simulink model "MatlabCode-Thermosys"  (R2014a)
settings: Solver=ode23tb  StartTime=0.0  StopTime=1000  RelTol=1e-3
libraries: thermosys x4
settings Model: CovSFcnEnable=on  Creator=garrow2  LastModifiedBy=VILLAVI1
settings DataIOCC: LimitDataPoints=off  SaveFormat=StructureWithTime
settings DebuggingCC: MergeDetectMultiDrivingBlocksExec=error  SolverPrmCheckMsg=none  FrameProcessingCompatibilityMsg=error
settings HardwareCC: ProdBitPerPointer=64  ProdLargestAtomicFloat=Float  ProdIntDivRoundTo=Zero  ProdEndianess=LittleEndian  ProdHWDeviceType=Specified
settings ModelReferenceCC: PropagateSignalLabelsOutOfModel=on

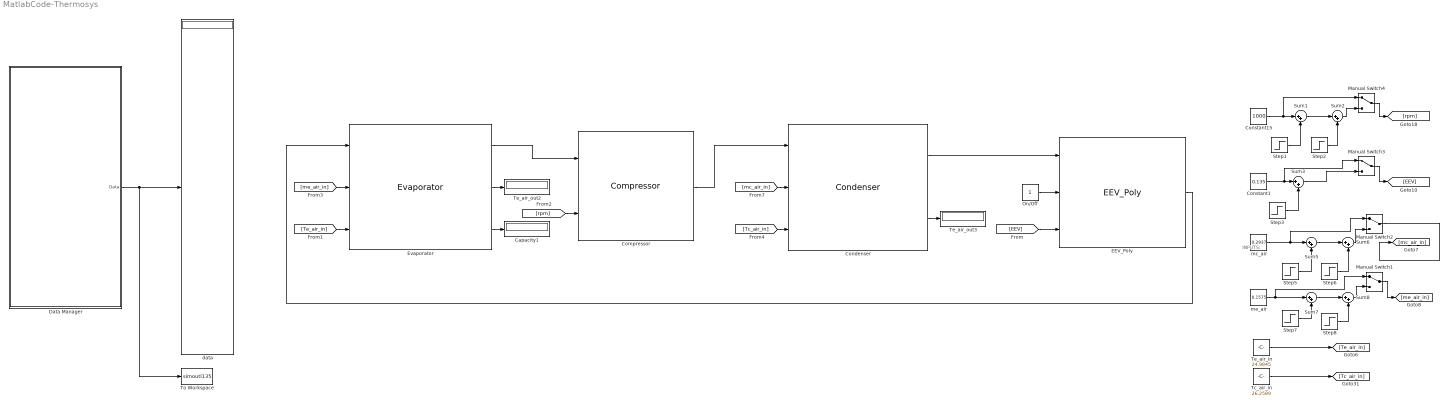
== system MatlabCode-Thermosys ==
  note: INPUTS:
  Capacity1 : Display
  Compressor : thermosys/Components/Compressor  Vk=3.042e-5  HTC=25  CFile=CompProp  REFR=R134a  Pk_ri=279.1497  Pk_ro=968.3655  Tk_ri=19.9747  Tk_ro=61.4005  mdot=0.0062  rpm=1500  IODS=Text
  Condenser : thermosys/Components/Condenser  Dh=8.1026e-3  L=10.6895  N=1  Ac_air=.089798964  As_air=2.792665382  As_ref=0.274993  Ac_ref=5.15631e-5  M_wall=4.65636  Cp_wall=.0467  PAF_TP=1  PAF_SH=0.5  PAF_SC=1  PAF_AIR=1.2  REFR=R134a  MFR=0.0062  PREF=968  RIT=61.8  ROE=250  MFA=0.2937  AIT=25  IODS=Text
  Constant1 : Constant  Value=0.135
  Constant15 : Constant  Value=1000
  Data Manager : Subsystem  AncestorBlock=thermosys/Support Components/Data Manager  mask{null=0}
      mask init:
      | set_param(gcb, 'LinkStatus', 'inactive')    % disable the library link
      settings: OpenFcn=data_manager
      mask Display: str ='Compressor/P_out_ref\nCompressor/h_out_ref\nCompressor/mdot_out_ref\nCondenser/P_out_ref\nCondenser/h_out_ref\nCondenser/T_out_ref\nCondenser/mdot_out_ref\nCondenser/T_out_air\nCondenser/T_wall1\nCondenser/T_wall2\nCondenser/T_wall3\nCondenser/Zeta1\nCondenser/Zeta2\nCondenser/Zeta3\nCondenser/Mass\nEEV_Poly/P_out_ref\nEEV_Poly/h_out_ref\nEEV_Poly/mdot_out_ref\nEvaporator/P_out_ref\nEvaporator/h_out_ref\nEvaporator/T_out_ref\nEvaporator/mdot_out_ref\nEvaporator/T_out_air\nEvaporator/T_wall1\nEvaporator/T_wall2\nEvaporator/Zeta1\nEvaporator/Zeta2\nEvaporator/Mass\nEvaporator/Cool_Cap'; fprintf(str)
  EEV_Poly : thermosys/Components/EEV_Poly  cv_max=4e-5  stroke_fraction=[0:0.1:1]  cv_fraction=[0:0.1:1].*(2.0-[0:0.1:1])  IODS=Text  REFR=R134a  p1=-2e-13  p2=5.6e-13  p3=-5.8e-13  p4=2.6e-13  p5=-1  p6=2  p7=1.1e-16
  Evaporator : thermosys/Components/Evaporator  Dh=8.126e-3  L=11.45794  N=1  Ac_air=.058384399  As_air=3.068019456  As_ref=.0291662649  Ac_ref=5.15631e-5  M_wall=2.7438213  Cp_wall=0.48772265  PAF_TP=1  PAF_SH=2  PAF_AIR=1.1  REFR=R134a  MFR=0.0062  PREF=295.3  HREFIN=245  TRO=12  MFA=0.105  AIT=25  IODS=Text
  Manual Switch{1..4} (4 alike) : ManualSwitch
  On/Off : Constant
  Step1 : Step  Time=100  After=-1500  SampleTime=0
  Step2 : Step  Time=500  After=1500  SampleTime=0
  Step3 : Step  Time=100  After=-0.06  SampleTime=0
  Step5 : Step  Time=100  After=-0.2937  SampleTime=0
  Step6 : Step  Time=500  After=0.2937  SampleTime=0
  Step7 : Step  Time=100  After=-0.105  SampleTime=0
  Step8 : Step  Time=500  After=0.105  SampleTime=0
  Sum{1..3,5..8} (7 alike) : Sum  Inputs=|++
  Tc_air_in : Constant  Value=26.2589
  Te_air_in : Constant  Value=24.9845
  Te_air_out2 : Display
  Te_air_out3 : Display
  To Workspace : ToWorkspace  VariableName=simoutl135  SaveFormat=Timeseries  SampleTime=-1
  data : Display
  mc_air : Constant  Value=0.2937
  me_air : Constant  Value=0.1575
  wires:
  [EEV] -> EEV_Poly/3
  On/Off/1 -> EEV_Poly/2
  [Tc_air_in] -> Condenser/3
  [mc_air_in] -> Condenser/2
  [rpm] -> Compressor/2
  [me_air_in] -> Evaporator/2
  [Te_air_in] -> Evaporator/3
  Evaporator/2 -> Te_air_out2/1
  Evaporator/3 -> Capacity1/1
  Condenser/2 -> Te_air_out3/1
  Evaporator/1 -> Compressor/1
  Compressor/1 -> Condenser/1
  Condenser/1 -> EEV_Poly/1
  EEV_Poly/1 -> Evaporator/1
  Tc_air_in/1 -> [Tc_air_in]
  Te_air_in/1 -> [Te_air_in]
  Constant15/1 -> Manual Switch4/1, Sum1/1
  Step1/1 -> Sum1/2
  Sum1/1 -> Sum2/1
  Step2/1 -> Sum2/2
  Constant1/1 -> Manual Switch3/1, Sum3/1
  Step3/1 -> Sum3/2
  Step5/1 -> Sum5/2
  Step6/1 -> Sum6/2
  mc_air/1 -> Manual Switch2/1, Sum5/1
  Sum5/1 -> Sum6/1
  Step7/1 -> Sum7/2
  Step8/1 -> Sum8/2
  Sum7/1 -> Sum8/1
  me_air/1 -> Manual Switch1/1, Sum7/1
  Sum6/1 -> Manual Switch2/2
  Data Manager/1(Data) -> To Workspace/1, data/1
  Sum8/1 -> Manual Switch1/2
  Manual Switch1/1 -> [me_air_in]
  Manual Switch2/1 -> [mc_air_in]
  Manual Switch3/1 -> [EEV]
  Manual Switch4/1 -> [rpm]
  Sum2/1 -> Manual Switch4/2
  Sum3/1 -> Manual Switch3/2

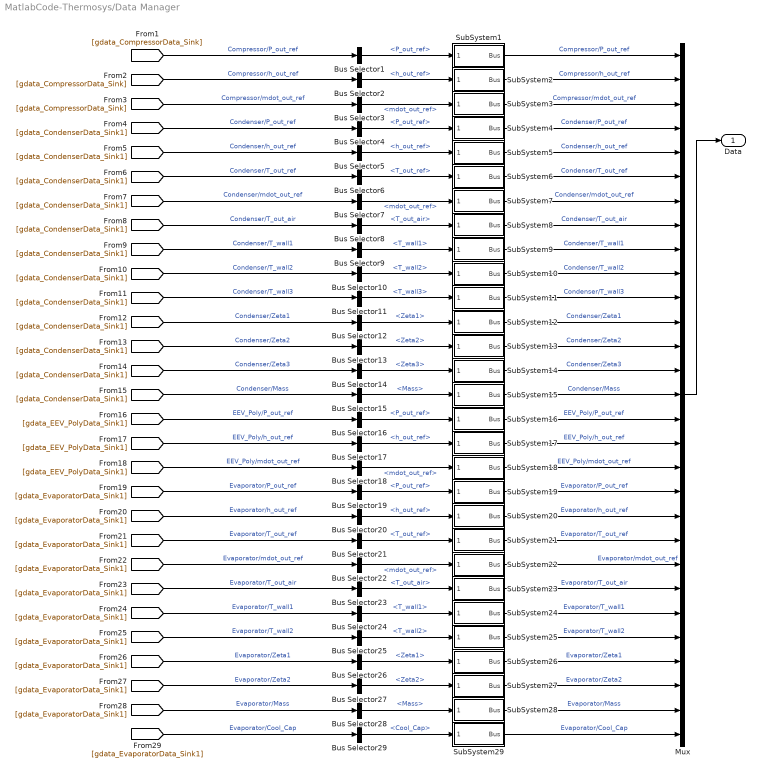
== system MatlabCode-Thermosys/Data Manager ==
  Bus Selector{1,4,16,19} (4 alike) : BusSelector  OutputSignals=P_out_ref
  Bus Selector10 : BusSelector  OutputSignals=T_wall2
  Bus Selector11 : BusSelector  OutputSignals=T_wall3
  Bus Selector12 : BusSelector  OutputSignals=Zeta1
  Bus Selector13 : BusSelector  OutputSignals=Zeta2
  Bus Selector14 : BusSelector  OutputSignals=Zeta3
  Bus Selector15 : BusSelector  OutputSignals=Mass
  Bus Selector{2,5,17,20} (4 alike) : BusSelector  OutputSignals=h_out_ref
  Bus Selector{3,7,18,22} (4 alike) : BusSelector  OutputSignals=mdot_out_ref
  Bus Selector21 : BusSelector  OutputSignals=T_out_ref
  Bus Selector23 : BusSelector  OutputSignals=T_out_air
  Bus Selector24 : BusSelector  OutputSignals=T_wall1
  Bus Selector25 : BusSelector  OutputSignals=T_wall2
  Bus Selector26 : BusSelector  OutputSignals=Zeta1
  Bus Selector27 : BusSelector  OutputSignals=Zeta2
  Bus Selector28 : BusSelector  OutputSignals=Mass
  Bus Selector29 : BusSelector  OutputSignals=Cool_Cap
  Bus Selector6 : BusSelector  OutputSignals=T_out_ref
  Bus Selector8 : BusSelector  OutputSignals=T_out_air
  Bus Selector9 : BusSelector  OutputSignals=T_wall1
  Mux : Mux  Inputs=29
  SubSystem1 : Subsystem
  SubSystem10 : Subsystem
  SubSystem11 : Subsystem
  SubSystem12 : Subsystem
  SubSystem13 : Subsystem
  SubSystem14 : Subsystem
  SubSystem15 : Subsystem
  SubSystem16 : Subsystem
  SubSystem17 : Subsystem
  SubSystem18 : Subsystem
  SubSystem19 : Subsystem
  SubSystem2 : Subsystem
  SubSystem20 : Subsystem
  SubSystem21 : Subsystem
  SubSystem22 : Subsystem
  SubSystem23 : Subsystem
  SubSystem24 : Subsystem
  SubSystem25 : Subsystem
  SubSystem26 : Subsystem
  SubSystem27 : Subsystem
  SubSystem28 : Subsystem
  SubSystem29 : Subsystem
  SubSystem3 : Subsystem
  SubSystem4 : Subsystem
  SubSystem5 : Subsystem
  SubSystem6 : Subsystem
  SubSystem7 : Subsystem
  SubSystem8 : Subsystem
  SubSystem9 : Subsystem
  Data : Outport
  wires:
  Mux/1 -> Data/1
  [gdata_CompressorData_Sink] -> Bus Selector1/1  "Compressor/P_out_ref"
  Bus Selector1/1 -> SubSystem1/1(Rename)  "<P_out_ref>"
  SubSystem1/1(Bus) -> Mux/1  "Compressor/P_out_ref"
  [gdata_CompressorData_Sink] -> Bus Selector2/1  "Compressor/h_out_ref"
  Bus Selector2/1 -> SubSystem2/1(Rename)  "<h_out_ref>"
  SubSystem2/1(Bus) -> Mux/2  "Compressor/h_out_ref"
  [gdata_CompressorData_Sink] -> Bus Selector3/1  "Compressor/mdot_out_ref"
  Bus Selector3/1 -> SubSystem3/1(Rename)  "<mdot_out_ref>"
  SubSystem3/1(Bus) -> Mux/3  "Compressor/mdot_out_ref"
  [gdata_CondenserData_Sink1] -> Bus Selector4/1  "Condenser/P_out_ref"
  Bus Selector4/1 -> SubSystem4/1(Rename)  "<P_out_ref>"
  SubSystem4/1(Bus) -> Mux/4  "Condenser/P_out_ref"
  [gdata_CondenserData_Sink1] -> Bus Selector5/1  "Condenser/h_out_ref"
  Bus Selector5/1 -> SubSystem5/1(Rename)  "<h_out_ref>"
  SubSystem5/1(Bus) -> Mux/5  "Condenser/h_out_ref"
  [gdata_CondenserData_Sink1] -> Bus Selector6/1  "Condenser/T_out_ref"
  Bus Selector6/1 -> SubSystem6/1(Rename)  "<T_out_ref>"
  SubSystem6/1(Bus) -> Mux/6  "Condenser/T_out_ref"
  [gdata_CondenserData_Sink1] -> Bus Selector7/1  "Condenser/mdot_out_ref"
  Bus Selector7/1 -> SubSystem7/1(Rename)  "<mdot_out_ref>"
  SubSystem7/1(Bus) -> Mux/7  "Condenser/mdot_out_ref"
  [gdata_CondenserData_Sink1] -> Bus Selector8/1  "Condenser/T_out_air"
  Bus Selector8/1 -> SubSystem8/1(Rename)  "<T_out_air>"
  SubSystem8/1(Bus) -> Mux/8  "Condenser/T_out_air"
  [gdata_CondenserData_Sink1] -> Bus Selector9/1  "Condenser/T_wall1"
  Bus Selector9/1 -> SubSystem9/1(Rename)  "<T_wall1>"
  SubSystem9/1(Bus) -> Mux/9  "Condenser/T_wall1"
  [gdata_CondenserData_Sink1] -> Bus Selector10/1  "Condenser/T_wall2"
  Bus Selector10/1 -> SubSystem10/1(Rename)  "<T_wall2>"
  SubSystem10/1(Bus) -> Mux/10  "Condenser/T_wall2"
  [gdata_CondenserData_Sink1] -> Bus Selector11/1  "Condenser/T_wall3"
  Bus Selector11/1 -> SubSystem11/1(Rename)  "<T_wall3>"
  SubSystem11/1(Bus) -> Mux/11  "Condenser/T_wall3"
  [gdata_CondenserData_Sink1] -> Bus Selector12/1  "Condenser/Zeta1"
  Bus Selector12/1 -> SubSystem12/1(Rename)  "<Zeta1>"
  SubSystem12/1(Bus) -> Mux/12  "Condenser/Zeta1"
  [gdata_CondenserData_Sink1] -> Bus Selector13/1  "Condenser/Zeta2"
  Bus Selector13/1 -> SubSystem13/1(Rename)  "<Zeta2>"
  SubSystem13/1(Bus) -> Mux/13  "Condenser/Zeta2"
  [gdata_CondenserData_Sink1] -> Bus Selector14/1  "Condenser/Zeta3"
  Bus Selector14/1 -> SubSystem14/1(Rename)  "<Zeta3>"
  SubSystem14/1(Bus) -> Mux/14  "Condenser/Zeta3"
  [gdata_CondenserData_Sink1] -> Bus Selector15/1  "Condenser/Mass"
  Bus Selector15/1 -> SubSystem15/1(Rename)  "<Mass>"
  SubSystem15/1(Bus) -> Mux/15  "Condenser/Mass"
  [gdata_EEV_PolyData_Sink1] -> Bus Selector16/1  "EEV_Poly/P_out_ref"
  Bus Selector16/1 -> SubSystem16/1(Rename)  "<P_out_ref>"
  SubSystem16/1(Bus) -> Mux/16  "EEV_Poly/P_out_ref"
  [gdata_EEV_PolyData_Sink1] -> Bus Selector17/1  "EEV_Poly/h_out_ref"
  Bus Selector17/1 -> SubSystem17/1(Rename)  "<h_out_ref>"
  SubSystem17/1(Bus) -> Mux/17  "EEV_Poly/h_out_ref"
  [gdata_EEV_PolyData_Sink1] -> Bus Selector18/1  "EEV_Poly/mdot_out_ref"
  Bus Selector18/1 -> SubSystem18/1(Rename)  "<mdot_out_ref>"
  SubSystem18/1(Bus) -> Mux/18  "EEV_Poly/mdot_out_ref"
  [gdata_EvaporatorData_Sink1] -> Bus Selector19/1  "Evaporator/P_out_ref"
  Bus Selector19/1 -> SubSystem19/1(Rename)  "<P_out_ref>"
  SubSystem19/1(Bus) -> Mux/19  "Evaporator/P_out_ref"
  [gdata_EvaporatorData_Sink1] -> Bus Selector20/1  "Evaporator/h_out_ref"
  Bus Selector20/1 -> SubSystem20/1(Rename)  "<h_out_ref>"
  SubSystem20/1(Bus) -> Mux/20  "Evaporator/h_out_ref"
  [gdata_EvaporatorData_Sink1] -> Bus Selector21/1  "Evaporator/T_out_ref"
  Bus Selector21/1 -> SubSystem21/1(Rename)  "<T_out_ref>"
  SubSystem21/1(Bus) -> Mux/21  "Evaporator/T_out_ref"
  [gdata_EvaporatorData_Sink1] -> Bus Selector22/1  "Evaporator/mdot_out_ref"
  Bus Selector22/1 -> SubSystem22/1(Rename)  "<mdot_out_ref>"
  SubSystem22/1(Bus) -> Mux/22  "Evaporator/mdot_out_ref"
  [gdata_EvaporatorData_Sink1] -> Bus Selector23/1  "Evaporator/T_out_air"
  Bus Selector23/1 -> SubSystem23/1(Rename)  "<T_out_air>"
  SubSystem23/1(Bus) -> Mux/23  "Evaporator/T_out_air"
  [gdata_EvaporatorData_Sink1] -> Bus Selector24/1  "Evaporator/T_wall1"
  Bus Selector24/1 -> SubSystem24/1(Rename)  "<T_wall1>"
  SubSystem24/1(Bus) -> Mux/24  "Evaporator/T_wall1"
  [gdata_EvaporatorData_Sink1] -> Bus Selector25/1  "Evaporator/T_wall2"
  Bus Selector25/1 -> SubSystem25/1(Rename)  "<T_wall2>"
  SubSystem25/1(Bus) -> Mux/25  "Evaporator/T_wall2"
  [gdata_EvaporatorData_Sink1] -> Bus Selector26/1  "Evaporator/Zeta1"
  Bus Selector26/1 -> SubSystem26/1(Rename)  "<Zeta1>"
  SubSystem26/1(Bus) -> Mux/26  "Evaporator/Zeta1"
  [gdata_EvaporatorData_Sink1] -> Bus Selector27/1  "Evaporator/Zeta2"
  Bus Selector27/1 -> SubSystem27/1(Rename)  "<Zeta2>"
  SubSystem27/1(Bus) -> Mux/27  "Evaporator/Zeta2"
  [gdata_EvaporatorData_Sink1] -> Bus Selector28/1  "Evaporator/Mass"
  Bus Selector28/1 -> SubSystem28/1(Rename)  "<Mass>"
  SubSystem28/1(Bus) -> Mux/28  "Evaporator/Mass"
  [gdata_EvaporatorData_Sink1] -> Bus Selector29/1  "Evaporator/Cool_Cap"
  Bus Selector29/1 -> SubSystem29/1(Rename)  "<Cool_Cap>"
  SubSystem29/1(Bus) -> Mux/29  "Evaporator/Cool_Cap"

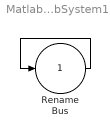
== system MatlabCode-Thermosys/Data Manager/SubSystem1 ==
  Rename : Inport
  Bus : Outport
  wires:
  Rename/1 -> Bus/1

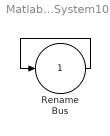
== system MatlabCode-Thermosys/Data Manager/SubSystem10 ==
  Rename : Inport
  Bus : Outport
  wires:
  Rename/1 -> Bus/1

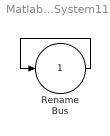
== system MatlabCode-Thermosys/Data Manager/SubSystem11 ==
  Rename : Inport
  Bus : Outport
  wires:
  Rename/1 -> Bus/1

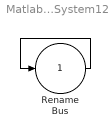
== system MatlabCode-Thermosys/Data Manager/SubSystem12 ==
  Rename : Inport
  Bus : Outport
  wires:
  Rename/1 -> Bus/1

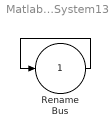
== system MatlabCode-Thermosys/Data Manager/SubSystem13 ==
  Rename : Inport
  Bus : Outport
  wires:
  Rename/1 -> Bus/1

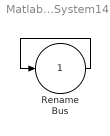
== system MatlabCode-Thermosys/Data Manager/SubSystem14 ==
  Rename : Inport
  Bus : Outport
  wires:
  Rename/1 -> Bus/1

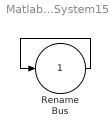
== system MatlabCode-Thermosys/Data Manager/SubSystem15 ==
  Rename : Inport
  Bus : Outport
  wires:
  Rename/1 -> Bus/1

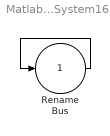
== system MatlabCode-Thermosys/Data Manager/SubSystem16 ==
  Rename : Inport
  Bus : Outport
  wires:
  Rename/1 -> Bus/1

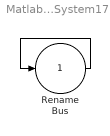
== system MatlabCode-Thermosys/Data Manager/SubSystem17 ==
  Rename : Inport
  Bus : Outport
  wires:
  Rename/1 -> Bus/1

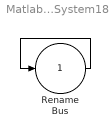
== system MatlabCode-Thermosys/Data Manager/SubSystem18 ==
  Rename : Inport
  Bus : Outport
  wires:
  Rename/1 -> Bus/1

== system MatlabCode-Thermosys/Data Manager/SubSystem19 ==
  Rename : Inport
  Bus : Outport
  wires:
  Rename/1 -> Bus/1

== system MatlabCode-Thermosys/Data Manager/SubSystem2 ==
  Rename : Inport
  Bus : Outport
  wires:
  Rename/1 -> Bus/1

== system MatlabCode-Thermosys/Data Manager/SubSystem20 ==
  Rename : Inport
  Bus : Outport
  wires:
  Rename/1 -> Bus/1

== system MatlabCode-Thermosys/Data Manager/SubSystem21 ==
  Rename : Inport
  Bus : Outport
  wires:
  Rename/1 -> Bus/1

== system MatlabCode-Thermosys/Data Manager/SubSystem22 ==
  Rename : Inport
  Bus : Outport
  wires:
  Rename/1 -> Bus/1

== system MatlabCode-Thermosys/Data Manager/SubSystem23 ==
  Rename : Inport
  Bus : Outport
  wires:
  Rename/1 -> Bus/1

== system MatlabCode-Thermosys/Data Manager/SubSystem24 ==
  Rename : Inport
  Bus : Outport
  wires:
  Rename/1 -> Bus/1

== system MatlabCode-Thermosys/Data Manager/SubSystem25 ==
  Rename : Inport
  Bus : Outport
  wires:
  Rename/1 -> Bus/1

== system MatlabCode-Thermosys/Data Manager/SubSystem26 ==
  Rename : Inport
  Bus : Outport
  wires:
  Rename/1 -> Bus/1

== system MatlabCode-Thermosys/Data Manager/SubSystem27 ==
  Rename : Inport
  Bus : Outport
  wires:
  Rename/1 -> Bus/1

== system MatlabCode-Thermosys/Data Manager/SubSystem28 ==
  Rename : Inport
  Bus : Outport
  wires:
  Rename/1 -> Bus/1

== system MatlabCode-Thermosys/Data Manager/SubSystem29 ==
  Rename : Inport
  Bus : Outport
  wires:
  Rename/1 -> Bus/1

== system MatlabCode-Thermosys/Data Manager/SubSystem3 ==
  Rename : Inport
  Bus : Outport
  wires:
  Rename/1 -> Bus/1

== system MatlabCode-Thermosys/Data Manager/SubSystem4 ==
  Rename : Inport
  Bus : Outport
  wires:
  Rename/1 -> Bus/1

== system MatlabCode-Thermosys/Data Manager/SubSystem5 ==
  Rename : Inport
  Bus : Outport
  wires:
  Rename/1 -> Bus/1

== system MatlabCode-Thermosys/Data Manager/SubSystem6 ==
  Rename : Inport
  Bus : Outport
  wires:
  Rename/1 -> Bus/1

== system MatlabCode-Thermosys/Data Manager/SubSystem7 ==
  Rename : Inport
  Bus : Outport
  wires:
  Rename/1 -> Bus/1

== system MatlabCode-Thermosys/Data Manager/SubSystem8 ==
  Rename : Inport
  Bus : Outport
  wires:
  Rename/1 -> Bus/1

== system MatlabCode-Thermosys/Data Manager/SubSystem9 ==
  Rename : Inport
  Bus : Outport
  wires:
  Rename/1 -> Bus/1
